simulink model "environment_model"  (Simulink 8.7)
settings: Solver=ode45  StartTime=0.0  StopTime=20000  MaxStep=1  RelTol=1e-3  AbsTol=1e-6
values from neighbouring files (symbols this model uses):
  initial_r = [7028000 0 0]    [constants.m]
  initial_v = [0 -1048 7458]    [constants.m]
  k = input(1)    [MagTorq.m]    (also in main.m = gain_range(i))
  Sat_I = [0.0506 0 0; 0 0.0506 0; 0 0 0.010]    [constants.m]
libraries: vrlib x1
settings Model: Creator=menjkim  LastModifiedBy=fy12jt
settings DataIOCC: InspectSignalLogs=on
settings OptimizationCC: ExpressionDepthLimit=2147483647
settings DebuggingCC: SolverPrmCheckMsg=warning  StateNameClashWarn=warning

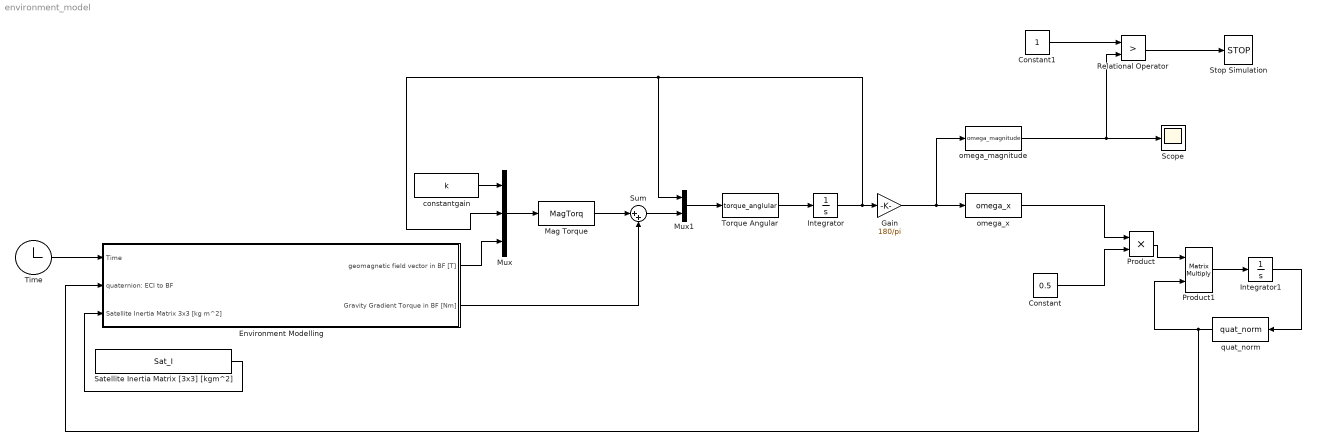
== system environment_model ==
  Constant : Constant  Value=0.5
  Constant1 : Constant
  Environment Modelling : Subsystem
  Gain : Gain  Gain=180/pi
  Integrator : Integrator  InitialCondition=[-0.1; 0.1; -0.2]
  Integrator1 : Integrator  InitialCondition=[0.1754; 0.5951; -0.7329; 0.2798]
  "Mag Torque " : MATLABFcn  MATLABFcn=MagTorq
  Mux : Mux  Inputs=3
  Mux1 : Mux  Inputs=2
  Product : Product
  Product1 : Product  Multiplication=Matrix(*)
  Relational Operator : RelationalOperator  Operator=>  OutDataTypeStr=boolean
  Satellite Inertia Matrix [3x3] [kgm^2] : Constant  Value=Sat_I
  Scope : Scope
  Stop Simulation : Stop
  Sum : Sum  Inputs=|++
  Time : Clock
      settings: Decimation=1000
  Torque Angular : MATLABFcn  MATLABFcn=torque_anglular
  constantgain : Constant  Value=k
  omega_magnitude : MATLABFcn  MATLABFcn=omega_magnitude
  omega_x : MATLABFcn  MATLABFcn=omega_x  Output1D=off
  "quat_norm " : MATLABFcn  MATLABFcn=quat_norm
  wires:
  Time/1 -> Environment Modelling/1(Time)
  Satellite Inertia Matrix [3x3] [kgm^2]/1 -> Environment Modelling/3(Satellite Inertia Matrix 3x3 [kg m^2])
  Environment Modelling/2(Gravity Gradient Torque in BF [Nm]) -> Sum/2
  Environment Modelling/1(geomagnetic field vector in BF [T]) -> Mux/3
  constantgain/1 -> Mux/1
  Mux/1 -> "Mag Torque "/1
  "Mag Torque "/1 -> Sum/1
  Sum/1 -> Mux1/2
  Mux1/1 -> Torque Angular/1
  Torque Angular/1 -> Integrator/1
  Integrator/1 -> Mux1/1, Mux/2, Gain/1
  Gain/1 -> omega_magnitude/1, omega_x/1
  omega_x/1 -> Product/1
  Constant/1 -> Product/2
  Product/1 -> Product1/1
  Product1/1 -> Integrator1/1
  omega_magnitude/1 -> Scope/1, Relational Operator/2
  Integrator1/1 -> "quat_norm "/1
  Relational Operator/1 -> Stop Simulation/1
  Constant1/1 -> Relational Operator/1
  "quat_norm "/1 -> Environment Modelling/2(quaternion: ECI to BF), Product1/2

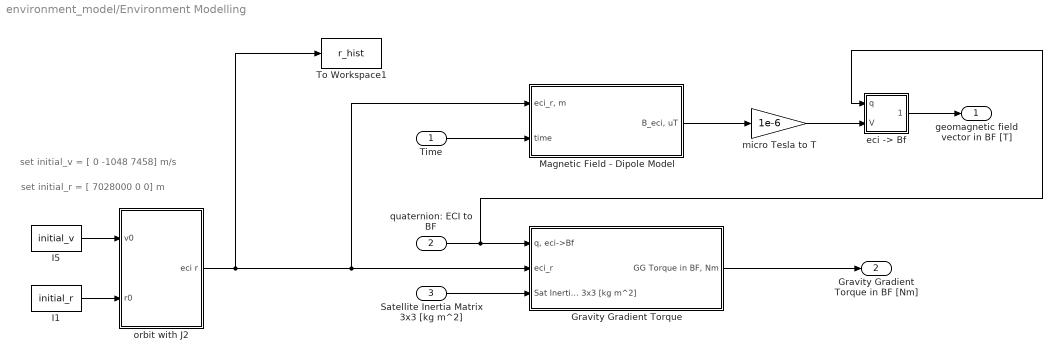
== system environment_model/Environment Modelling ==
  note: set initial_v = [ 0 -1048 7458] m/s
  note: set initial_r = [ 7028000 0 0] m
  Time : Inport
  quaternion: ECI to BF : Inport  Port=2
  Satellite Inertia Matrix 3x3 [kg m^2] : Inport  Port=3
  Gravity Gradient Torque : Subsystem
  I1 : Constant  Value=initial_r
  I5 : Constant  Value=initial_v
  Magnetic Field - Dipole Model : Subsystem
  To Workspace1 : ToWorkspace  VariableName=r_hist  SampleTime=-1
  "eci -> Bf" : Subsystem  mask(Quaternion Vector Transform){}
      mask help:
      | Transforms a vector using a quaternion:
      |
      |     vout = (q*)(v)(q)
      |
      | The first input is the quaternion, the second input is the vector.
  micro Tesla to T : Gain  Gain=1e-6
  orbit with J2 : Subsystem
  geomagnetic field vector in BF [T] : Outport
  Gravity Gradient Torque in BF [Nm] : Outport  Port=2
  wires:
  orbit with J2/1(eci r) -> To Workspace1/1, Magnetic Field - Dipole Model/1("eci_r, m"), Gravity Gradient Torque/2(eci_r)
  Time/1 -> Magnetic Field - Dipole Model/2(time)
  quaternion: ECI to BF/1 -> "eci -> Bf"/1(q), Gravity Gradient Torque/1("q, eci->Bf")
  Magnetic Field - Dipole Model/1("B_eci, uT") -> micro Tesla to T/1
  micro Tesla to T/1 -> "eci -> Bf"/2(V)
  "eci -> Bf"/1(q*Vq) -> geomagnetic field vector in BF [T]/1
  Gravity Gradient Torque/1("GG Torque in BF, Nm") -> Gravity Gradient Torque in BF [Nm]/1
  Satellite Inertia Matrix 3x3 [kg m^2]/1 -> Gravity Gradient Torque/3(Sat Inertia 3x3 [kg m^2])
  I1/1 -> orbit with J2/2(r0)
  I5/1 -> orbit with J2/1(v0)

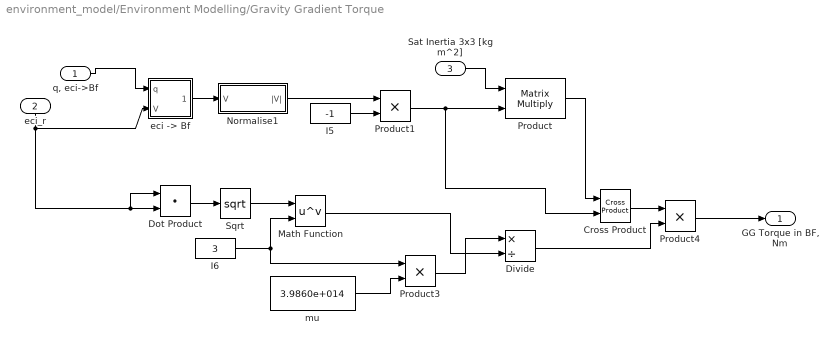
== system environment_model/Environment Modelling/Gravity Gradient Torque ==
  "q, eci->Bf" : Inport
  eci_r : Inport  Port=2
  Sat Inertia 3x3 [kg m^2] : Inport  Port=3
  Cross Product : vrlib/Utilities/Cross Product
  Divide : Product  Inputs=*/
  Dot Product : DotProduct  InputSameDT=on  OutDataTypeStr=Inherit: Inherit via internal rule
  I5 : Constant  Value=-1
  I6 : Constant  Value=3
  Math Function : Math  Operator=pow  SaturateOnIntegerOverflow=on
  Normalise1 : Subsystem
      mask help:
      | Normalise vector (Root-Sum-Squares = 1).
      | If magnitude of input vector is zero, then resultant output vector is also returned as zero.
      mask Display: disp('|V|')
  Product : Product  Multiplication=Matrix(*)  RndMeth=Zero
  Product1 : Product  RndMeth=Zero
  Product3 : Product  RndMeth=Zero
  Product4 : Product  RndMeth=Zero
  Sqrt : Math  Operator=sqrt  SaturateOnIntegerOverflow=on
  "eci -> Bf" : Subsystem  mask(Quaternion Vector Transform){}
      mask help:
      | Transforms a vector using a quaternion:
      |
      |     vout = (q*)(v)(q)
      |
      | The first input is the quaternion, the second input is the vector.
  mu : Constant  Value=3.9860e+014
  "GG Torque in BF, Nm" : Outport
  wires:
  Product4/1 -> "GG Torque in BF, Nm"/1
  eci_r/1 -> Dot Product/1, Dot Product/2, "eci -> Bf"/2(V)
  "q, eci->Bf"/1 -> "eci -> Bf"/1(q)
  Product3/1 -> Divide/1
  Divide/1 -> Product4/2
  mu/1 -> Product3/2
  Cross Product/1 -> Product4/1
  Product/1 -> Cross Product/1
  Math Function/1 -> Divide/2
  I6/1 -> Product3/1, Math Function/2
  Sqrt/1 -> Math Function/1
  Dot Product/1 -> Sqrt/1
  I5/1 -> Product1/2
  Product1/1 -> Cross Product/2, Product/2
  Sat Inertia 3x3 [kg m^2]/1 -> Product/1
  Normalise1/1(|V|) -> Product1/1
  "eci -> Bf"/1(q*Vq) -> Normalise1/1("V ")

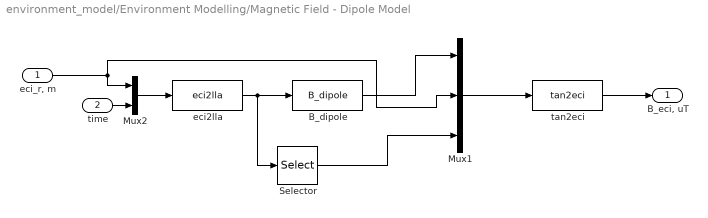
== system environment_model/Environment Modelling/Magnetic Field - Dipole Model ==
  "eci_r, m" : Inport
  time : Inport  Port=2
  B_dipole : MATLABFcn  MATLABFcn=B_dipole  OutputDimensions=3
  Mux1 : Mux  Inputs=3
  Mux2 : Mux  Inputs=2
  Selector : Selector  InputPortWidth=3  IndexOptions=Index vector (dialog)  Indices=[1]  OutputSizes=1
  eci2lla : MATLABFcn  MATLABFcn=eci2lla  OutputDimensions=3
  tan2eci : MATLABFcn  MATLABFcn=tan2eci  OutputDimensions=3
  "B_eci, uT" : Outport
  wires:
  eci2lla/1 -> Selector/1, B_dipole/1
  tan2eci/1 -> "B_eci, uT"/1
  Mux2/1 -> eci2lla/1
  time/1 -> Mux2/2
  "eci_r, m"/1 -> Mux1/2, Mux2/1
  B_dipole/1 -> Mux1/1
  Mux1/1 -> tan2eci/1
  Selector/1 -> Mux1/3

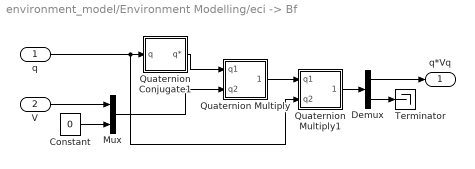
== system environment_model/Environment Modelling/eci -> Bf ==
  q : Inport  PortDimensions=4
  V : Inport  Port=2  PortDimensions=3
  Constant : Constant  Value=0
  Demux : Demux  Outputs=[3 1]
  Mux : Mux  Inputs=2
  Quaternion Conjugate1 : Subsystem  mask(Quaternion Conjugate){}
      mask help: q* = [ -q(1) -q(2) -q(3) q(4) ]
      mask Display: disp('q*')
  Quaternion Multiply : Subsystem  mask(Quaternion Multiply){}
      mask help: Multiplies input quaternions: qout = (q1)(q2)
  Quaternion Multiply1 : Subsystem  mask(Quaternion Multiply){}
      mask help: Multiplies input quaternions: qout = (q1)(q2)
  Terminator : Terminator
  q*Vq : Outport  InitialOutput=0
  wires:
  V/1 -> Mux/1
  Constant/1 -> Mux/2
  q/1 -> Quaternion Conjugate1/1(q), Quaternion Multiply1/2(q2)
  Quaternion Multiply1/1(q1q2) -> Demux/1
  Demux/2 -> Terminator/1
  Demux/1 -> q*Vq/1
  Mux/1 -> Quaternion Multiply/2(q2)
  Quaternion Conjugate1/1(q*) -> Quaternion Multiply/1(q1)
  Quaternion Multiply/1(q1q2) -> Quaternion Multiply1/1(q1)

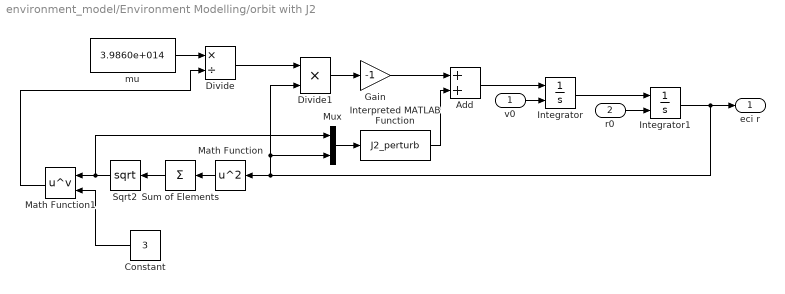
== system environment_model/Environment Modelling/orbit with J2 ==
  v0 : Inport
  r0 : Inport  Port=2
  Add : Sum
  Constant : Constant  Value=3
  Divide : Product  Inputs=*/
  Divide1 : Product  Inputs=**
  Gain : Gain  Gain=-1
  Integrator : Integrator  InitialConditionSource=external  InitialCondition=[-1021 -88 -7488]
  Integrator1 : Integrator  InitialConditionSource=external  InitialCondition=[596030 -6952400 0]
  Interpreted MATLAB Function : MATLABFcn  MATLABFcn=J2_perturb
  Math Function : Math  Operator=square  SaturateOnIntegerOverflow=on
  Math Function1 : Math  Operator=pow  SaturateOnIntegerOverflow=on
  Mux : Mux  Inputs=2
  Sqrt2 : Math  Operator=sqrt  SaturateOnIntegerOverflow=on
  Sum of Elements : Sum  Inputs=+
  mu : Constant  Value=3.9860e+014
  eci r : Outport
  wires:
  r0/1 -> Integrator1/2
  v0/1 -> Integrator/2
  Integrator1/1 -> eci r/1, Math Function/1, Divide1/2, Mux/2
  Integrator/1 -> Integrator1/1
  Sum of Elements/1 -> Sqrt2/1
  Math Function/1 -> Sum of Elements/1
  Divide1/1 -> Gain/1
  Divide/1 -> Divide1/1
  mu/1 -> Divide/1
  Sqrt2/1 -> Mux/1, Math Function1/1
  Math Function1/1 -> Divide/2
  Constant/1 -> Math Function1/2
  Gain/1 -> Add/1
  Add/1 -> Integrator/1
  Mux/1 -> Interpreted MATLAB Function/1
  Interpreted MATLAB Function/1 -> Add/2

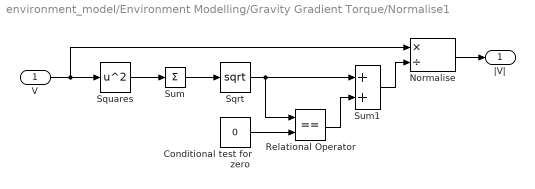
== system environment_model/Environment Modelling/Gravity Gradient Torque/Normalise1 ==
  "V " : Inport
  Conditional test for zero : Constant  Value=0
  Normalise : Product  Inputs=*/  SaturateOnIntegerOverflow=on  InputSameDT=on  OutDataTypeStr=Inherit: Same as first input
  Relational Operator : RelationalOperator  Operator===  OutDataTypeStr=float('double')
  Sqrt : Math  Operator=sqrt  SaturateOnIntegerOverflow=on
  Squares : Math  Operator=square  SaturateOnIntegerOverflow=on
  Sum : Sum  Inputs=1  SaturateOnIntegerOverflow=on  InputSameDT=on  OutDataTypeStr=Inherit: Same as first input
  Sum1 : Sum  SaturateOnIntegerOverflow=on
  |V| : Outport
  wires:
  Relational Operator/1 -> Sum1/2
  Sum1/1 -> Normalise/2
  Conditional test for zero/1 -> Relational Operator/2
  Normalise/1 -> |V|/1
  "V "/1 -> Squares/1, Normalise/1
  Squares/1 -> Sum/1
  Sum/1 -> Sqrt/1
  Sqrt/1 -> Sum1/1, Relational Operator/1

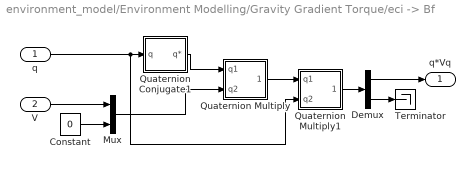
== system environment_model/Environment Modelling/Gravity Gradient Torque/eci -> Bf ==
  q : Inport  PortDimensions=4
  V : Inport  Port=2  PortDimensions=3
  Constant : Constant  Value=0
  Demux : Demux  Outputs=[3 1]
  Mux : Mux  Inputs=2
  Quaternion Conjugate1 : Subsystem  mask(Quaternion Conjugate){}
      mask help: q* = [ -q(1) -q(2) -q(3) q(4) ]
      mask Display: disp('q*')
  Quaternion Multiply : Subsystem  mask(Quaternion Multiply){}
      mask help: Multiplies input quaternions: qout = (q1)(q2)
  Quaternion Multiply1 : Subsystem  mask(Quaternion Multiply){}
      mask help: Multiplies input quaternions: qout = (q1)(q2)
  Terminator : Terminator
  q*Vq : Outport  InitialOutput=0
  wires:
  Quaternion Multiply/1(q1q2) -> Quaternion Multiply1/1(q1)
  Quaternion Conjugate1/1(q*) -> Quaternion Multiply/1(q1)
  Mux/1 -> Quaternion Multiply/2(q2)
  Demux/1 -> q*Vq/1
  Demux/2 -> Terminator/1
  Quaternion Multiply1/1(q1q2) -> Demux/1
  q/1 -> Quaternion Multiply1/2(q2), Quaternion Conjugate1/1(q)
  Constant/1 -> Mux/2
  V/1 -> Mux/1

== system environment_model/Environment Modelling/eci -> Bf/Quaternion Conjugate1 ==
  q : Inport  PortDimensions=4
  Demux : Demux  Outputs=[3 1]
  Gain : Gain  Gain=-1  SaturateOnIntegerOverflow=on  OutDataTypeStr=Inherit: Same as input  ParamDataTypeStr=Inherit: Same as input
  Mux : Mux  Inputs=2
  q* : Outport  InitialOutput=0
  wires:
  q/1 -> Demux/1
  Demux/1 -> Gain/1  "[ q(1)  q(2)  q(3) ]"
  Gain/1 -> Mux/1
  Demux/2 -> Mux/2  "q(4)"
  Mux/1 -> q*/1

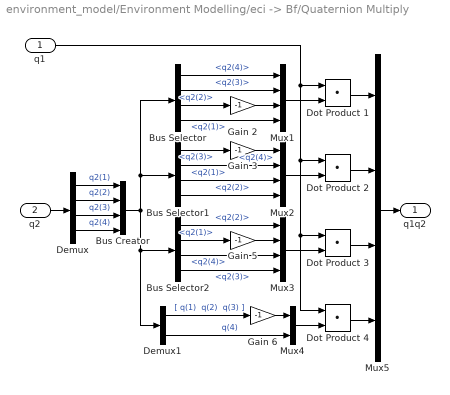
== system environment_model/Environment Modelling/eci -> Bf/Quaternion Multiply ==
  q1 : Inport  PortDimensions=4
  q2 : Inport  Port=2  PortDimensions=4
  Bus Creator : BusCreator  Inputs=4
  Bus Selector : BusSelector  OutputSignals=q2(4),q2(3),q2(2),q2(1)
  Bus Selector1 : BusSelector  OutputSignals=q2(3),q2(4),q2(1),q2(2)
  Bus Selector2 : BusSelector  OutputSignals=q2(2),q2(1),q2(4),q2(3)
  Demux : Demux
  Demux1 : Demux  Outputs=[3 1]
  Dot Product {1..4} (4 alike) : DotProduct  InputSameDT=on  OutDataTypeStr=Inherit: Inherit via internal rule
  Gain {2..3,5..6} (4 alike) : Gain  Gain=-1  SaturateOnIntegerOverflow=on  OutDataTypeStr=Inherit: Same as input  ParamDataTypeStr=Inherit: Same as input
  Mux{1..3,5} (4 alike) : Mux
  Mux4 : Mux  Inputs=2
  q1q2 : Outport  InitialOutput=0
  wires:
  Demux1/2 -> Mux4/2  "q(4)"
  Gain 6/1 -> Mux4/1
  Demux1/1 -> Gain 6/1  "[ q(1)  q(2)  q(3) ]"
  Mux4/1 -> Dot Product 4/2
  Bus Selector2/4 -> Mux3/4  "<q2(3)>"
  Bus Selector2/1 -> Mux3/1  "<q2(2)>"
  Gain 5/1 -> Mux3/2
  Bus Selector2/2 -> Gain 5/1  "<q2(1)>"
  Bus Selector1/4 -> Mux2/4  "<q2(2)>"
  Bus Selector1/3 -> Mux2/3  "<q2(1)>"
  Gain 3/1 -> Mux2/1
  Bus Selector1/1 -> Gain 3/1  "<q2(3)>"
  Bus Selector/4 -> Mux1/4  "<q2(1)>"
  Gain 2/1 -> Mux1/3
  Bus Selector/3 -> Gain 2/1  "<q2(2)>"
  Bus Selector/2 -> Mux1/2  "<q2(3)>"
  Bus Selector/1 -> Mux1/1  "<q2(4)>"
  Bus Selector1/2 -> Mux2/2  "<q2(4)>"
  Bus Selector2/3 -> Mux3/3  "<q2(4)>"
  Mux1/1 -> Dot Product 1/2
  Mux2/1 -> Dot Product 2/2
  Mux3/1 -> Dot Product 3/2
  q1/1 -> Dot Product 1/1, Dot Product 2/1, Dot Product 3/1, Dot Product 4/1
  Dot Product 1/1 -> Mux5/1
  Dot Product 3/1 -> Mux5/3
  Dot Product 4/1 -> Mux5/4
  Mux5/1 -> q1q2/1
  Dot Product 2/1 -> Mux5/2
  Bus Creator/1 -> Demux1/1, Bus Selector2/1, Bus Selector/1, Bus Selector1/1
  q2/1 -> Demux/1
  Demux/1 -> Bus Creator/1  "q2(1)"
  Demux/2 -> Bus Creator/2  "q2(2)"
  Demux/3 -> Bus Creator/3  "q2(3)"
  Demux/4 -> Bus Creator/4  "q2(4)"

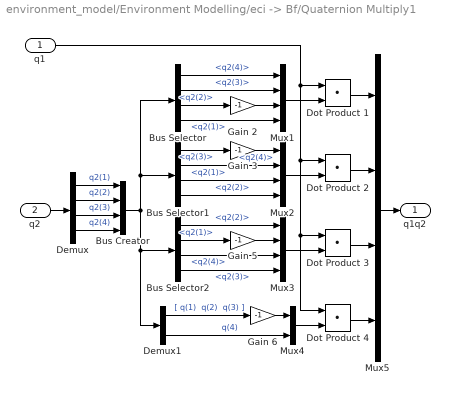
== system environment_model/Environment Modelling/eci -> Bf/Quaternion Multiply1 ==
  q1 : Inport  PortDimensions=4
  q2 : Inport  Port=2  PortDimensions=4
  Bus Creator : BusCreator  Inputs=4
  Bus Selector : BusSelector  OutputSignals=q2(4),q2(3),q2(2),q2(1)
  Bus Selector1 : BusSelector  OutputSignals=q2(3),q2(4),q2(1),q2(2)
  Bus Selector2 : BusSelector  OutputSignals=q2(2),q2(1),q2(4),q2(3)
  Demux : Demux
  Demux1 : Demux  Outputs=[3 1]
  Dot Product {1..4} (4 alike) : DotProduct  InputSameDT=on  OutDataTypeStr=Inherit: Inherit via internal rule
  Gain {2..3,5..6} (4 alike) : Gain  Gain=-1  SaturateOnIntegerOverflow=on  OutDataTypeStr=Inherit: Same as input  ParamDataTypeStr=Inherit: Same as input
  Mux{1..3,5} (4 alike) : Mux
  Mux4 : Mux  Inputs=2
  q1q2 : Outport  InitialOutput=0
  wires:
  Demux1/2 -> Mux4/2  "q(4)"
  Gain 6/1 -> Mux4/1
  Demux1/1 -> Gain 6/1  "[ q(1)  q(2)  q(3) ]"
  Mux4/1 -> Dot Product 4/2
  Bus Selector2/4 -> Mux3/4  "<q2(3)>"
  Bus Selector2/1 -> Mux3/1  "<q2(2)>"
  Gain 5/1 -> Mux3/2
  Bus Selector2/2 -> Gain 5/1  "<q2(1)>"
  Bus Selector1/4 -> Mux2/4  "<q2(2)>"
  Bus Selector1/3 -> Mux2/3  "<q2(1)>"
  Gain 3/1 -> Mux2/1
  Bus Selector1/1 -> Gain 3/1  "<q2(3)>"
  Bus Selector/4 -> Mux1/4  "<q2(1)>"
  Gain 2/1 -> Mux1/3
  Bus Selector/3 -> Gain 2/1  "<q2(2)>"
  Bus Selector/2 -> Mux1/2  "<q2(3)>"
  Bus Selector/1 -> Mux1/1  "<q2(4)>"
  Bus Selector1/2 -> Mux2/2  "<q2(4)>"
  Bus Selector2/3 -> Mux3/3  "<q2(4)>"
  Mux1/1 -> Dot Product 1/2
  Mux2/1 -> Dot Product 2/2
  Mux3/1 -> Dot Product 3/2
  q1/1 -> Dot Product 1/1, Dot Product 2/1, Dot Product 3/1, Dot Product 4/1
  Dot Product 1/1 -> Mux5/1
  Dot Product 3/1 -> Mux5/3
  Dot Product 4/1 -> Mux5/4
  Mux5/1 -> q1q2/1
  Dot Product 2/1 -> Mux5/2
  Bus Creator/1 -> Demux1/1, Bus Selector2/1, Bus Selector/1, Bus Selector1/1
  q2/1 -> Demux/1
  Demux/1 -> Bus Creator/1  "q2(1)"
  Demux/2 -> Bus Creator/2  "q2(2)"
  Demux/3 -> Bus Creator/3  "q2(3)"
  Demux/4 -> Bus Creator/4  "q2(4)"

== system environment_model/Environment Modelling/Gravity Gradient Torque/eci -> Bf/Quaternion Conjugate1 ==
  q : Inport  PortDimensions=4
  Demux : Demux  Outputs=[3 1]
  Gain : Gain  Gain=-1  SaturateOnIntegerOverflow=on  OutDataTypeStr=Inherit: Same as input  ParamDataTypeStr=Inherit: Same as input
  Mux : Mux  Inputs=2
  q* : Outport  InitialOutput=0
  wires:
  Mux/1 -> q*/1
  Demux/2 -> Mux/2  "q(4)"
  Gain/1 -> Mux/1
  Demux/1 -> Gain/1  "[ q(1)  q(2)  q(3) ]"
  q/1 -> Demux/1

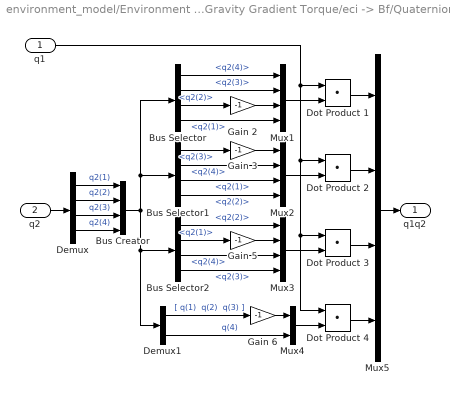
== system environment_model/Environment Modelling/Gravity Gradient Torque/eci -> Bf/Quaternion Multiply ==
  q1 : Inport  PortDimensions=4
  q2 : Inport  Port=2  PortDimensions=4
  Bus Creator : BusCreator  Inputs=4
  Bus Selector : BusSelector  OutputSignals=q2(4),q2(3),q2(2),q2(1)
  Bus Selector1 : BusSelector  OutputSignals=q2(3),q2(4),q2(1),q2(2)
  Bus Selector2 : BusSelector  OutputSignals=q2(2),q2(1),q2(4),q2(3)
  Demux : Demux
  Demux1 : Demux  Outputs=[3 1]
  Dot Product {1..4} (4 alike) : DotProduct  InputSameDT=on  OutDataTypeStr=Inherit: Inherit via internal rule
  Gain {2..3,5..6} (4 alike) : Gain  Gain=-1  SaturateOnIntegerOverflow=on  OutDataTypeStr=Inherit: Same as input  ParamDataTypeStr=Inherit: Same as input
  Mux{1..3,5} (4 alike) : Mux
  Mux4 : Mux  Inputs=2
  q1q2 : Outport  InitialOutput=0
  wires:
  Demux/4 -> Bus Creator/4  "q2(4)"
  Demux/3 -> Bus Creator/3  "q2(3)"
  Demux/2 -> Bus Creator/2  "q2(2)"
  Demux/1 -> Bus Creator/1  "q2(1)"
  q2/1 -> Demux/1
  Bus Creator/1 -> Bus Selector1/1, Bus Selector/1, Bus Selector2/1, Demux1/1
  Dot Product 2/1 -> Mux5/2
  Mux5/1 -> q1q2/1
  Dot Product 4/1 -> Mux5/4
  Dot Product 3/1 -> Mux5/3
  Dot Product 1/1 -> Mux5/1
  q1/1 -> Dot Product 4/1, Dot Product 3/1, Dot Product 2/1, Dot Product 1/1
  Mux3/1 -> Dot Product 3/2
  Mux2/1 -> Dot Product 2/2
  Mux1/1 -> Dot Product 1/2
  Bus Selector2/3 -> Mux3/3  "<q2(4)>"
  Bus Selector1/2 -> Mux2/2  "<q2(4)>"
  Bus Selector/1 -> Mux1/1  "<q2(4)>"
  Bus Selector/2 -> Mux1/2  "<q2(3)>"
  Bus Selector/3 -> Gain 2/1  "<q2(2)>"
  Gain 2/1 -> Mux1/3
  Bus Selector/4 -> Mux1/4  "<q2(1)>"
  Bus Selector1/1 -> Gain 3/1  "<q2(3)>"
  Gain 3/1 -> Mux2/1
  Bus Selector1/3 -> Mux2/3  "<q2(1)>"
  Bus Selector1/4 -> Mux2/4  "<q2(2)>"
  Bus Selector2/2 -> Gain 5/1  "<q2(1)>"
  Gain 5/1 -> Mux3/2
  Bus Selector2/1 -> Mux3/1  "<q2(2)>"
  Bus Selector2/4 -> Mux3/4  "<q2(3)>"
  Mux4/1 -> Dot Product 4/2
  Demux1/1 -> Gain 6/1  "[ q(1)  q(2)  q(3) ]"
  Gain 6/1 -> Mux4/1
  Demux1/2 -> Mux4/2  "q(4)"

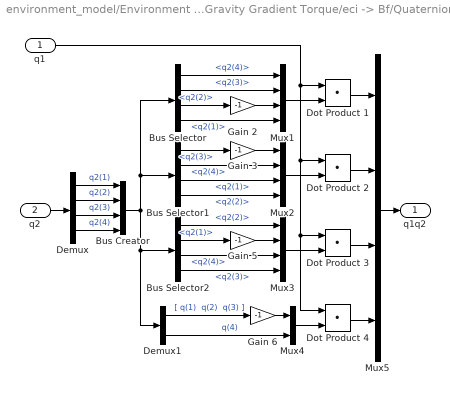
== system environment_model/Environment Modelling/Gravity Gradient Torque/eci -> Bf/Quaternion Multiply1 ==
  q1 : Inport  PortDimensions=4
  q2 : Inport  Port=2  PortDimensions=4
  Bus Creator : BusCreator  Inputs=4
  Bus Selector : BusSelector  OutputSignals=q2(4),q2(3),q2(2),q2(1)
  Bus Selector1 : BusSelector  OutputSignals=q2(3),q2(4),q2(1),q2(2)
  Bus Selector2 : BusSelector  OutputSignals=q2(2),q2(1),q2(4),q2(3)
  Demux : Demux
  Demux1 : Demux  Outputs=[3 1]
  Dot Product {1..4} (4 alike) : DotProduct  InputSameDT=on  OutDataTypeStr=Inherit: Inherit via internal rule
  Gain {2..3,5..6} (4 alike) : Gain  Gain=-1  SaturateOnIntegerOverflow=on  OutDataTypeStr=Inherit: Same as input  ParamDataTypeStr=Inherit: Same as input
  Mux{1..3,5} (4 alike) : Mux
  Mux4 : Mux  Inputs=2
  q1q2 : Outport  InitialOutput=0
  wires:
  Demux/4 -> Bus Creator/4  "q2(4)"
  Demux/3 -> Bus Creator/3  "q2(3)"
  Demux/2 -> Bus Creator/2  "q2(2)"
  Demux/1 -> Bus Creator/1  "q2(1)"
  q2/1 -> Demux/1
  Bus Creator/1 -> Bus Selector1/1, Bus Selector/1, Bus Selector2/1, Demux1/1
  Dot Product 2/1 -> Mux5/2
  Mux5/1 -> q1q2/1
  Dot Product 4/1 -> Mux5/4
  Dot Product 3/1 -> Mux5/3
  Dot Product 1/1 -> Mux5/1
  q1/1 -> Dot Product 4/1, Dot Product 3/1, Dot Product 2/1, Dot Product 1/1
  Mux3/1 -> Dot Product 3/2
  Mux2/1 -> Dot Product 2/2
  Mux1/1 -> Dot Product 1/2
  Bus Selector2/3 -> Mux3/3  "<q2(4)>"
  Bus Selector1/2 -> Mux2/2  "<q2(4)>"
  Bus Selector/1 -> Mux1/1  "<q2(4)>"
  Bus Selector/2 -> Mux1/2  "<q2(3)>"
  Bus Selector/3 -> Gain 2/1  "<q2(2)>"
  Gain 2/1 -> Mux1/3
  Bus Selector/4 -> Mux1/4  "<q2(1)>"
  Bus Selector1/1 -> Gain 3/1  "<q2(3)>"
  Gain 3/1 -> Mux2/1
  Bus Selector1/3 -> Mux2/3  "<q2(1)>"
  Bus Selector1/4 -> Mux2/4  "<q2(2)>"
  Bus Selector2/2 -> Gain 5/1  "<q2(1)>"
  Gain 5/1 -> Mux3/2
  Bus Selector2/1 -> Mux3/1  "<q2(2)>"
  Bus Selector2/4 -> Mux3/4  "<q2(3)>"
  Mux4/1 -> Dot Product 4/2
  Demux1/1 -> Gain 6/1  "[ q(1)  q(2)  q(3) ]"
  Gain 6/1 -> Mux4/1
  Demux1/2 -> Mux4/2  "q(4)"
